simulink model "quadcopter_final"  (R2017a)
settings: Solver=VariableStepAuto  StartTime=0.0  StopTime=100  RelTol=1e-3
model workspace (MAT data in the model file):
  Izz = 0.019
values from neighbouring files (symbols this model uses):
  Ax = 0.1    [quadcopter_final.mat]
  Ay = 0.1    [quadcopter_final.mat]
  Az = 0    [quadcopter_final.mat]
  b = 3.59e-05    [quadcopter_final.mat]
  d = 2.081e-06    [quadcopter_final.mat]
  g = 9.8    [quadcopter_final.mat]
  Ixx = 0.00963    [quadcopter_final.mat]
  Iyy = 0.0096    [quadcopter_final.mat]
  Jr = 0.04439    [quadcopter_final.mat]
  l = 0.24    [quadcopter_final.mat]
  m = 0.9928    [quadcopter_final.mat]
libraries: simulink x5
settings Model: Creator=Sarthak  LastModifiedBy=Sarthak

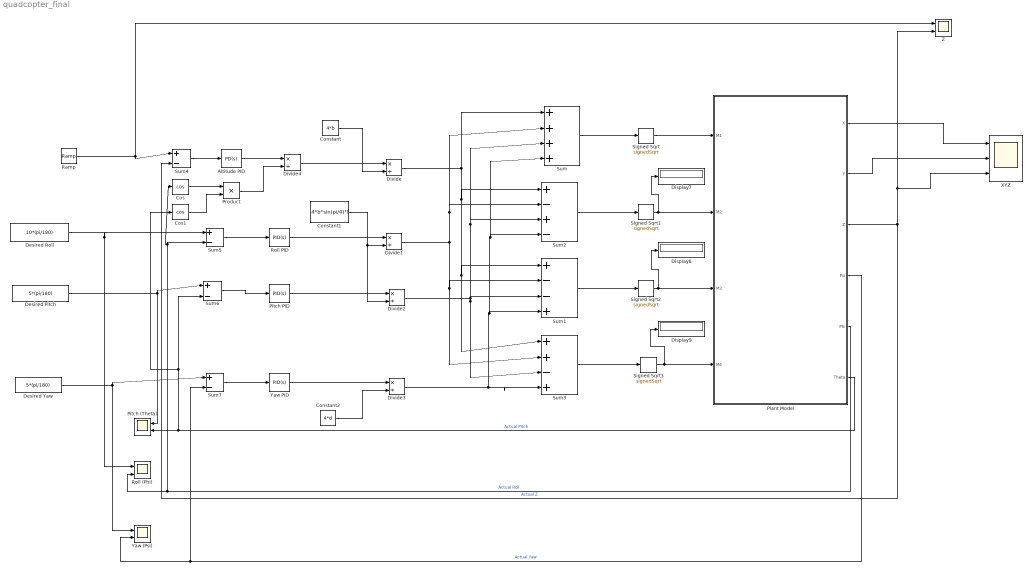
== system quadcopter_final ==
  Altitude PID : simulink/Continuous/PID Controller  Controller=PD  TimeDomain=Continuous-time  SampleTime=-1  IntegratorMethod=Forward Euler  FilterMethod=Forward Euler  Form=Parallel  UseFilter=on  ControllerParametersSource=internal  P=4  I=0.1  D=2  N=1  InitialConditionSource=internal  InitialConditionForIntegrator=0  InitialConditionForFilter=0  ExternalReset=none  LimitOutput=off  UpperSaturationLimit=inf  LowerSaturationLimit=-inf  LinearizeAsGain=on  AntiWindupMode=none  Kb=1  TrackingMode=off  Kt=1  PParamMin=[]  PParamMax=[]  IParamMin=[]  IParamMax=[]  DParamMin=[]  DParamMax=[]  NParamMin=[]  NParamMax=[]  KbParamMin=[]  KbParamMax=[]  KtParamMin=[]  KtParamMax=[]  POutMin=[]  POutMax=[]  IOutMin=[]  IOutMax=[]  DOutMin=[]  DOutMax=[]  NOutMin=[]  NOutMax=[]  KbOutMin=[]  KbOutMax=[]  KtOutMin=[]  KtOutMax=[]  IntegratorOutMin=[]  IntegratorOutMax=[]  FilterOutMin=[]  FilterOutMax=[]  SumOutMin=[]  SumOutMax=[]  SumI1OutMin=[]  SumI1OutMax=[]  SumI2OutMin=[]  SumI2OutMax=[]  SumI3OutMin=[]  SumI3OutMax=[]  SumDOutMin=[]  SumDOutMax=[]  SaturationOutMin=[]  SaturationOutMax=[]  IntegratorContinuousStateAttributes=''  IntegratorStateMustResolveToSignalObject=off  IntegratorRTWStateStorageClass=Auto  FilterContinuousStateAttributes=''  FilterStateMustResolveToSignalObject=off  FilterRTWStateStorageClass=Auto  DifferentiatorICPrevScaledInput=0  DifferentiatorOutMin=[]  DifferentiatorOutMax=[]  InitialConditionSetting=State (most efficient)
  Constant : Constant  Value=4*b
  Constant1 : Constant  Value=4*b*sin(pi/4)*l
  Constant2 : Constant  Value=4*d
  Cos : Trigonometry  Operator=cos
  Cos1 : Trigonometry  Operator=cos
  Desired Pitch : Constant  Value=5*(pi/180)
  Desired Roll : Constant  Value=10*(pi/180)
  Desired Yaw : Constant  Value=5*(pi/180)
  Display7 : Display
  Display8 : Display
  Display9 : Display
  Divide{,1..4} (5 alike) : Product  Inputs=*/
  Pitch (Theta) : Scope  NumInputPorts=2
  Pitch PID : simulink/Continuous/PID Controller  Controller=PID  TimeDomain=Continuous-time  SampleTime=-1  IntegratorMethod=Forward Euler  FilterMethod=Forward Euler  Form=Parallel  UseFilter=on  ControllerParametersSource=internal  P=1e-3  I=1e-5  D=1e-2  N=1  InitialConditionSource=internal  InitialConditionForIntegrator=0  InitialConditionForFilter=0  ExternalReset=none  LimitOutput=off  UpperSaturationLimit=inf  LowerSaturationLimit=-inf  LinearizeAsGain=on  AntiWindupMode=none  Kb=1  TrackingMode=off  Kt=1  PParamMin=[]  PParamMax=[]  IParamMin=[]  IParamMax=[]  DParamMin=[]  DParamMax=[]  NParamMin=[]  NParamMax=[]  KbParamMin=[]  KbParamMax=[]  KtParamMin=[]  KtParamMax=[]  POutMin=[]  POutMax=[]  IOutMin=[]  IOutMax=[]  DOutMin=[]  DOutMax=[]  NOutMin=[]  NOutMax=[]  KbOutMin=[]  KbOutMax=[]  KtOutMin=[]  KtOutMax=[]  IntegratorOutMin=[]  IntegratorOutMax=[]  FilterOutMin=[]  FilterOutMax=[]  SumOutMin=[]  SumOutMax=[]  SumI1OutMin=[]  SumI1OutMax=[]  SumI2OutMin=[]  SumI2OutMax=[]  SumI3OutMin=[]  SumI3OutMax=[]  SumDOutMin=[]  SumDOutMax=[]  SaturationOutMin=[]  SaturationOutMax=[]  IntegratorContinuousStateAttributes=''  IntegratorStateMustResolveToSignalObject=off  IntegratorRTWStateStorageClass=Auto  FilterContinuousStateAttributes=''  FilterStateMustResolveToSignalObject=off  FilterRTWStateStorageClass=Auto  DifferentiatorICPrevScaledInput=0  DifferentiatorOutMin=[]  DifferentiatorOutMax=[]  InitialConditionSetting=State (most efficient)
  Plant Model : Subsystem
  Product : Product
  Ramp : simulink/Sources/Ramp  slope=1  start=0  X0=0
  Roll (Phi) : Scope  NumInputPorts=2
  Roll PID : simulink/Continuous/PID Controller  Controller=PID  TimeDomain=Continuous-time  SampleTime=-1  IntegratorMethod=Forward Euler  FilterMethod=Forward Euler  Form=Parallel  UseFilter=on  ControllerParametersSource=internal  P=1e-3  I=2.45847996540361e-05  D=1  N=100  InitialConditionSource=internal  InitialConditionForIntegrator=0  InitialConditionForFilter=0  ExternalReset=none  LimitOutput=off  UpperSaturationLimit=inf  LowerSaturationLimit=-inf  LinearizeAsGain=on  AntiWindupMode=none  Kb=1  TrackingMode=off  Kt=1  PParamMin=[]  PParamMax=[]  IParamMin=[]  IParamMax=[]  DParamMin=[]  DParamMax=[]  NParamMin=[]  NParamMax=[]  KbParamMin=[]  KbParamMax=[]  KtParamMin=[]  KtParamMax=[]  POutMin=[]  POutMax=[]  IOutMin=[]  IOutMax=[]  DOutMin=[]  DOutMax=[]  NOutMin=[]  NOutMax=[]  KbOutMin=[]  KbOutMax=[]  KtOutMin=[]  KtOutMax=[]  IntegratorOutMin=[]  IntegratorOutMax=[]  FilterOutMin=[]  FilterOutMax=[]  SumOutMin=[]  SumOutMax=[]  SumI1OutMin=[]  SumI1OutMax=[]  SumI2OutMin=[]  SumI2OutMax=[]  SumI3OutMin=[]  SumI3OutMax=[]  SumDOutMin=[]  SumDOutMax=[]  SaturationOutMin=[]  SaturationOutMax=[]  IntegratorContinuousStateAttributes=''  IntegratorStateMustResolveToSignalObject=off  IntegratorRTWStateStorageClass=Auto  FilterContinuousStateAttributes=''  FilterStateMustResolveToSignalObject=off  FilterRTWStateStorageClass=Auto  DifferentiatorICPrevScaledInput=0  DifferentiatorOutMin=[]  DifferentiatorOutMax=[]  InitialConditionSetting=State (most efficient)
  Signed Sqrt{,1..3} (4 alike) : Sqrt  Operator=signedSqrt  SaturateOnIntegerOverflow=on
  Sum : Sum  Inputs=|++++
  Sum1 : Sum  Inputs=|+--+
  Sum2 : Sum  Inputs=|+-+-
  Sum3 : Sum  Inputs=|++-+
  Sum{4..7} (4 alike) : Sum  Inputs=|+-
  XYZ : Scope  NumInputPorts=3
  Yaw (Psi) : Scope  NumInputPorts=2
  Yaw PID : simulink/Continuous/PID Controller  Controller=PID  TimeDomain=Continuous-time  SampleTime=-1  IntegratorMethod=Forward Euler  FilterMethod=Forward Euler  Form=Parallel  UseFilter=on  ControllerParametersSource=internal  P=1e-3  I=1e-5  D=0.5e-2  N=1  InitialConditionSource=internal  InitialConditionForIntegrator=0  InitialConditionForFilter=0  ExternalReset=none  LimitOutput=off  UpperSaturationLimit=inf  LowerSaturationLimit=-inf  LinearizeAsGain=on  AntiWindupMode=none  Kb=1  TrackingMode=off  Kt=1  PParamMin=[]  PParamMax=[]  IParamMin=[]  IParamMax=[]  DParamMin=[]  DParamMax=[]  NParamMin=[]  NParamMax=[]  KbParamMin=[]  KbParamMax=[]  KtParamMin=[]  KtParamMax=[]  POutMin=[]  POutMax=[]  IOutMin=[]  IOutMax=[]  DOutMin=[]  DOutMax=[]  NOutMin=[]  NOutMax=[]  KbOutMin=[]  KbOutMax=[]  KtOutMin=[]  KtOutMax=[]  IntegratorOutMin=[]  IntegratorOutMax=[]  FilterOutMin=[]  FilterOutMax=[]  SumOutMin=[]  SumOutMax=[]  SumI1OutMin=[]  SumI1OutMax=[]  SumI2OutMin=[]  SumI2OutMax=[]  SumI3OutMin=[]  SumI3OutMax=[]  SumDOutMin=[]  SumDOutMax=[]  SaturationOutMin=[]  SaturationOutMax=[]  IntegratorContinuousStateAttributes=''  IntegratorStateMustResolveToSignalObject=off  IntegratorRTWStateStorageClass=Auto  FilterContinuousStateAttributes=''  FilterStateMustResolveToSignalObject=off  FilterRTWStateStorageClass=Auto  DifferentiatorICPrevScaledInput=0  DifferentiatorOutMin=[]  DifferentiatorOutMax=[]  InitialConditionSetting=State (most efficient)
  Z : Scope  NumInputPorts=2
  wires:
  Signed Sqrt/1 -> Plant Model/1(M1)
  Signed Sqrt1/1 -> Display7/1, Plant Model/2(M2)
  Signed Sqrt2/1 -> Display8/1, Plant Model/3(M3)
  Signed Sqrt3/1 -> Display9/1, Plant Model/4(M4)
  Sum/1 -> Signed Sqrt/1
  Sum2/1 -> Signed Sqrt1/1
  Sum1/1 -> Signed Sqrt2/1
  Sum3/1 -> Signed Sqrt3/1
  Divide/1 -> Sum3/1, Sum1/1, Sum2/1, Sum/1
  Divide1/1 -> Sum/2, Sum2/2, Sum3/2, Sum1/2
  Divide2/1 -> Sum3/3, Sum1/3, Sum2/3, Sum/3
  Divide3/1 -> Sum/4, Sum2/4, Sum1/4, Sum3/4
  Constant/1 -> Divide/2
  Constant1/1 -> Divide2/2, Divide1/2
  Constant2/1 -> Divide3/2
  Divide4/1 -> Divide/1
  Altitude PID/1 -> Divide4/1
  Product/1 -> Divide4/2
  Cos/1 -> Product/1
  Cos1/1 -> Product/2
  Roll PID/1 -> Divide1/1
  Pitch PID/1 -> Divide2/1
  Yaw PID/1 -> Divide3/1
  Sum4/1 -> Altitude PID/1
  Sum5/1 -> Roll PID/1
  Sum6/1 -> Pitch PID/1
  Sum7/1 -> Yaw PID/1
  Desired Roll/1 -> Roll (Phi)/1, Sum5/1
  Desired Pitch/1 -> Sum6/1, Pitch (Theta)/1
  Desired Yaw/1 -> Sum7/1, Yaw (Psi)/1
  Ramp/1 -> Sum4/1, Z/1
  Plant Model/6(Theta) -> Cos1/1, Sum6/2, Pitch (Theta)/2  "Actual Pitch"
  Plant Model/5(Phi) -> Cos/1, Sum5/2, Roll (Phi)/2  "Actual Roll"
  Plant Model/4(Psi) -> Sum7/2, Yaw (Psi)/2  "Actual Yaw"
  Plant Model/3(Z) -> Sum4/2, XYZ/3, Z/2  "Actual Z"
  Plant Model/1(X) -> XYZ/1
  Plant Model/2(Y) -> XYZ/2

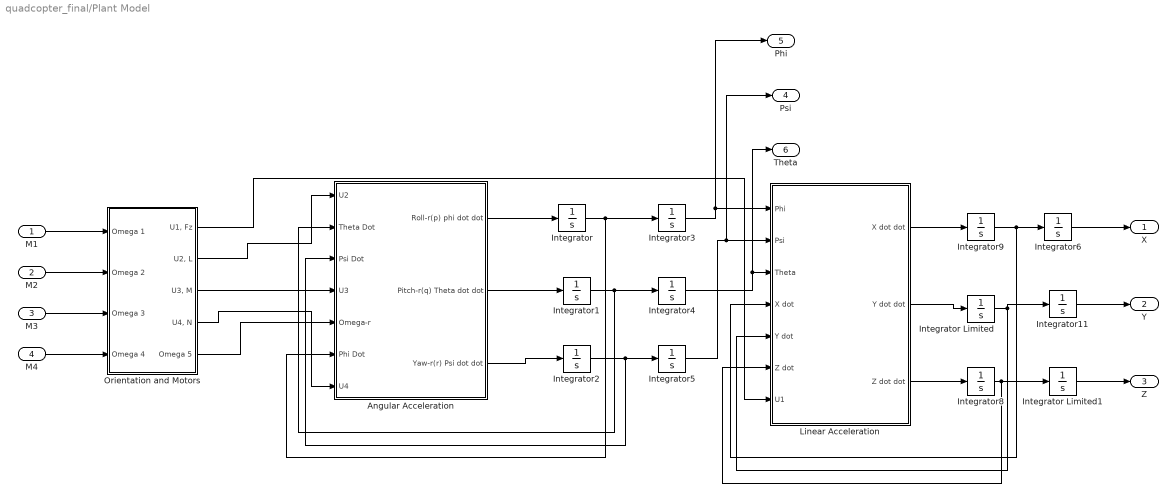
== system quadcopter_final/Plant Model ==
  M1 : Inport
  M2 : Inport  Port=2
  M3 : Inport  Port=3
  M4 : Inport  Port=4
  Angular Acceleration : Subsystem
  Integrator{,1..2,6,8..9,11} (7 alike) : Integrator
  Integrator Limited : Integrator  LimitOutput=on  LowerSaturationLimit=0
  Integrator Limited1 : Integrator  LimitOutput=on  LowerSaturationLimit=0
  Integrator3 : Integrator  WrapState=on
  Integrator4 : Integrator  WrapState=on
  Integrator5 : Integrator  WrapState=on
  Linear Acceleration : Subsystem
  Orientation and Motors : Subsystem
  X : Outport
  Y : Outport  Port=2
  Z : Outport  Port=3
  Psi : Outport  Port=4
  Phi : Outport  Port=5
  Theta : Outport  Port=6
  wires:
  M1/1 -> Orientation and Motors/1(Omega 1)
  M2/1 -> Orientation and Motors/2(Omega 2)
  M3/1 -> Orientation and Motors/3(Omega 3)
  M4/1 -> Orientation and Motors/4(Omega 4)
  Orientation and Motors/2("U2, L") -> Angular Acceleration/1(U2)
  Orientation and Motors/3("U3, M") -> Angular Acceleration/4(U3)
  Orientation and Motors/4("U4, N") -> Angular Acceleration/7(U4)
  Orientation and Motors/5(Omega 5) -> Angular Acceleration/5(Omega-r)
  Angular Acceleration/1(Roll-r(p) phi dot dot) -> Integrator/1
  Angular Acceleration/2(Pitch-r(q) Theta dot dot) -> Integrator1/1
  Angular Acceleration/3(Yaw-r(r) Psi dot dot) -> Integrator2/1
  Integrator/1 -> Angular Acceleration/6(Phi Dot), Integrator3/1
  Integrator2/1 -> Integrator5/1, Angular Acceleration/3(Psi Dot)
  Integrator3/1 -> Phi/1, Linear Acceleration/1(Phi)
  Integrator4/1 -> Theta/1, Linear Acceleration/3(Theta)
  Integrator5/1 -> Psi/1, Linear Acceleration/2(Psi)
  Integrator1/1 -> Integrator4/1, Angular Acceleration/2(Theta Dot)
  Orientation and Motors/1("U1, Fz") -> Linear Acceleration/7(U1)
  Integrator8/1 -> Integrator Limited1/1, Linear Acceleration/6(Z dot)
  Linear Acceleration/3(Z dot dot) -> Integrator8/1
  Linear Acceleration/2(Y dot dot) -> Integrator Limited/1
  Linear Acceleration/1(X dot dot) -> Integrator9/1
  Integrator9/1 -> Linear Acceleration/4(X dot), Integrator6/1
  Integrator Limited/1 -> Integrator11/1, Linear Acceleration/5(Y dot)
  Integrator Limited1/1 -> Z/1
  Integrator11/1 -> Y/1
  Integrator6/1 -> X/1

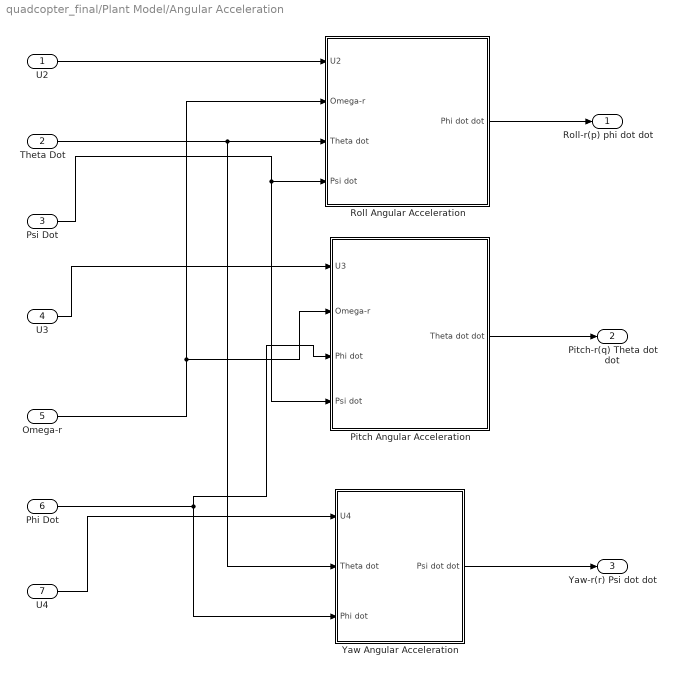
== system quadcopter_final/Plant Model/Angular Acceleration ==
  U2 : Inport
  Theta Dot : Inport  Port=2
  Psi Dot : Inport  Port=3
  U3 : Inport  Port=4
  Omega-r : Inport  Port=5
  Phi Dot : Inport  Port=6
  U4 : Inport  Port=7
  Pitch Angular Acceleration : Subsystem
  Roll Angular Acceleration : Subsystem
  Yaw Angular Acceleration : Subsystem
  Roll-r(p) phi dot dot : Outport
  Pitch-r(q) Theta dot dot : Outport  Port=2
  Yaw-r(r) Psi dot dot : Outport  Port=3
  wires:
  U2/1 -> Roll Angular Acceleration/1(U2)
  Omega-r/1 -> Pitch Angular Acceleration/2(Omega-r), Roll Angular Acceleration/2(Omega-r)
  Theta Dot/1 -> Yaw Angular Acceleration/2(Theta dot), Roll Angular Acceleration/3(Theta dot)
  Psi Dot/1 -> Pitch Angular Acceleration/4(Psi dot), Roll Angular Acceleration/4(Psi dot)
  U3/1 -> Pitch Angular Acceleration/1(U3)
  Phi Dot/1 -> Pitch Angular Acceleration/3(Phi dot), Yaw Angular Acceleration/3(Phi dot)
  U4/1 -> Yaw Angular Acceleration/1(U4)
  Roll Angular Acceleration/1(Phi dot dot) -> Roll-r(p) phi dot dot/1
  Pitch Angular Acceleration/1(Theta dot dot) -> Pitch-r(q) Theta dot dot/1
  Yaw Angular Acceleration/1(Psi dot dot) -> Yaw-r(r) Psi dot dot/1

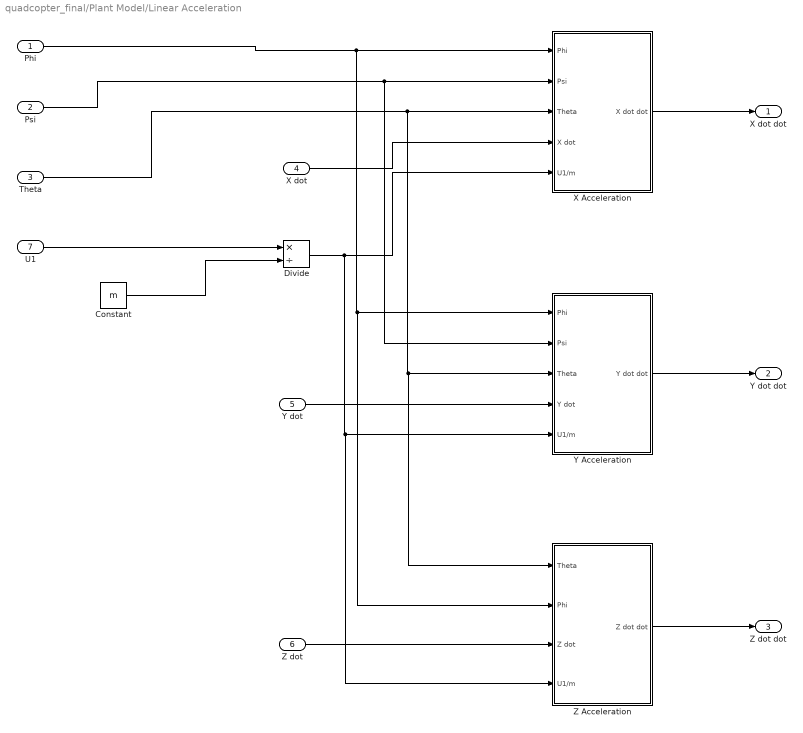
== system quadcopter_final/Plant Model/Linear Acceleration ==
  Phi : Inport
  Psi : Inport  Port=2
  Theta : Inport  Port=3
  X dot : Inport  Port=4
  Y dot : Inport  Port=5
  Z dot : Inport  Port=6
  U1 : Inport  Port=7
  Constant : Constant  Value=m
  Divide : Product  Inputs=*/
  X Acceleration : Subsystem
  Y Acceleration : Subsystem
  Z Acceleration : Subsystem
  X dot dot : Outport
  Y dot dot : Outport  Port=2
  Z dot dot : Outport  Port=3
  wires:
  Phi/1 -> Z Acceleration/2(Phi), Y Acceleration/1(Phi), X Acceleration/1(Phi)
  Psi/1 -> Y Acceleration/2(Psi), X Acceleration/2(Psi)
  Theta/1 -> Z Acceleration/1(Theta), Y Acceleration/3(Theta), X Acceleration/3(Theta)
  X dot/1 -> X Acceleration/4(X dot)
  Divide/1 -> Z Acceleration/4(U1/m), Y Acceleration/5(U1/m), X Acceleration/5(U1/m)
  U1/1 -> Divide/1
  Constant/1 -> Divide/2
  X Acceleration/1(X dot dot) -> X dot dot/1
  Y dot/1 -> Y Acceleration/4(Y dot)
  Y Acceleration/1(Y dot dot) -> Y dot dot/1
  Z dot/1 -> Z Acceleration/3(Z dot)
  Z Acceleration/1(Z dot dot) -> Z dot dot/1

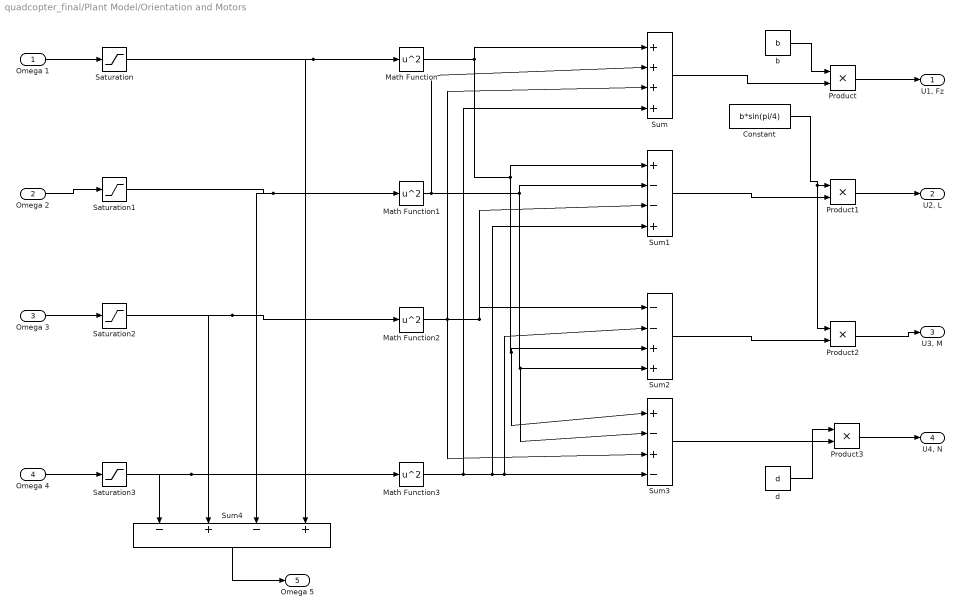
== system quadcopter_final/Plant Model/Orientation and Motors ==
  Omega 1 : Inport
  Omega 2 : Inport  Port=2
  Omega 3 : Inport  Port=3
  Omega 4 : Inport  Port=4
  Constant : Constant  Value=b*sin(pi/4)
  Math Function{,1..3} (4 alike) : Math  Operator=square  SaturateOnIntegerOverflow=on
  Product{,1..3} (4 alike) : Product
  Saturation{,1..3} (4 alike) : Saturate  UpperLimit=inf  LowerLimit=0
  Sum : Sum  Inputs=|++++
  Sum1 : Sum  Inputs=|+--+
  Sum2 : Sum  Inputs=|--++
  Sum3 : Sum  Inputs=|+-+-
  Sum4 : Sum  Inputs=|-+-+
  "b " : Constant  Value=b
  d : Constant  Value=d
  "U1, Fz" : Outport
  "U2, L" : Outport  Port=2
  "U3, M" : Outport  Port=3
  "U4, N" : Outport  Port=4
  Omega 5 : Outport  Port=5
  wires:
  Product/1 -> "U1, Fz"/1
  Product1/1 -> "U2, L"/1
  Product2/1 -> "U3, M"/1
  Product3/1 -> "U4, N"/1
  Sum/1 -> Product/2
  Sum1/1 -> Product1/2
  Sum2/1 -> Product2/2
  Sum3/1 -> Product3/2
  "b "/1 -> Product/1
  d/1 -> Product3/1
  Constant/1 -> Product1/1, Product2/1
  Math Function/1 -> Sum3/1, Sum2/3, Sum1/1, Sum/1
  Math Function1/1 -> Sum/2, Sum3/2, Sum2/4, Sum1/2
  Math Function2/1 -> Sum3/3, Sum/3, Sum1/3, Sum2/1
  Math Function3/1 -> Sum/4, Sum1/4, Sum2/2, Sum3/4
  Omega 1/1 -> Saturation/1
  Saturation/1 -> Sum4/4, Math Function/1
  Saturation1/1 -> Sum4/3, Math Function1/1
  Saturation2/1 -> Sum4/2, Math Function2/1
  Saturation3/1 -> Sum4/1, Math Function3/1
  Omega 4/1 -> Saturation3/1
  Omega 3/1 -> Saturation2/1
  Omega 2/1 -> Saturation1/1
  Sum4/1 -> Omega 5/1

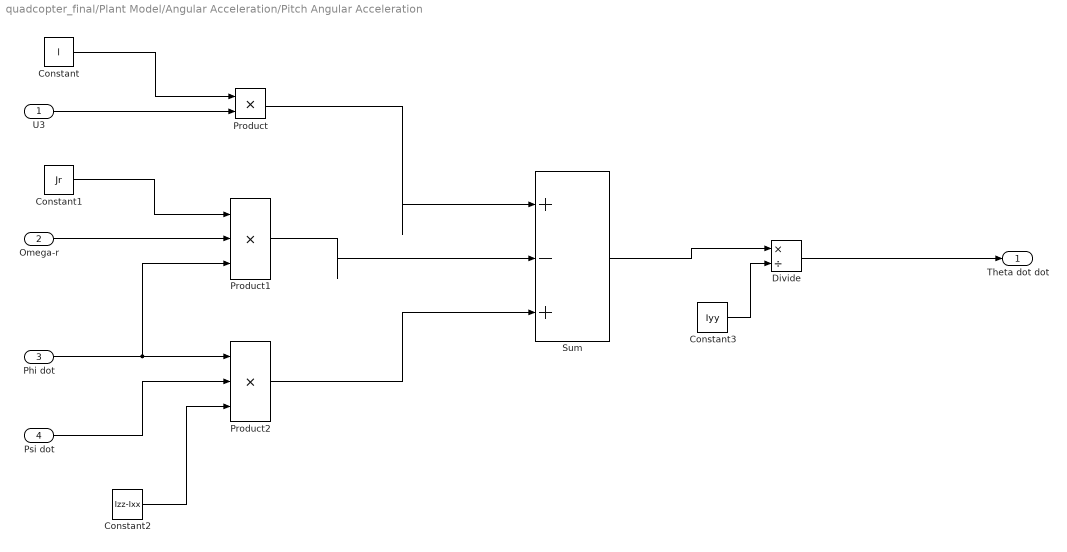
== system quadcopter_final/Plant Model/Angular Acceleration/Pitch Angular Acceleration ==
  U3 : Inport
  Omega-r : Inport  Port=2
  Phi dot : Inport  Port=3
  Psi dot : Inport  Port=4
  Constant : Constant  Value=l
  Constant1 : Constant  Value=Jr
  Constant2 : Constant  Value=Izz-Ixx
  Constant3 : Constant  Value=Iyy
  Divide : Product  Inputs=*/
  Product : Product
  Product1 : Product  Inputs=3
  Product2 : Product  Inputs=3
  Sum : Sum  Inputs=|+-+
  Theta dot dot : Outport
  wires:
  U3/1 -> Product/2
  Constant/1 -> Product/1
  Omega-r/1 -> Product1/2
  Constant1/1 -> Product1/1
  Phi dot/1 -> Product2/1, Product1/3
  Psi dot/1 -> Product2/2
  Constant2/1 -> Product2/3
  Product/1 -> Sum/1
  Product1/1 -> Sum/2
  Product2/1 -> Sum/3
  Sum/1 -> Divide/1
  Constant3/1 -> Divide/2
  Divide/1 -> Theta dot dot/1

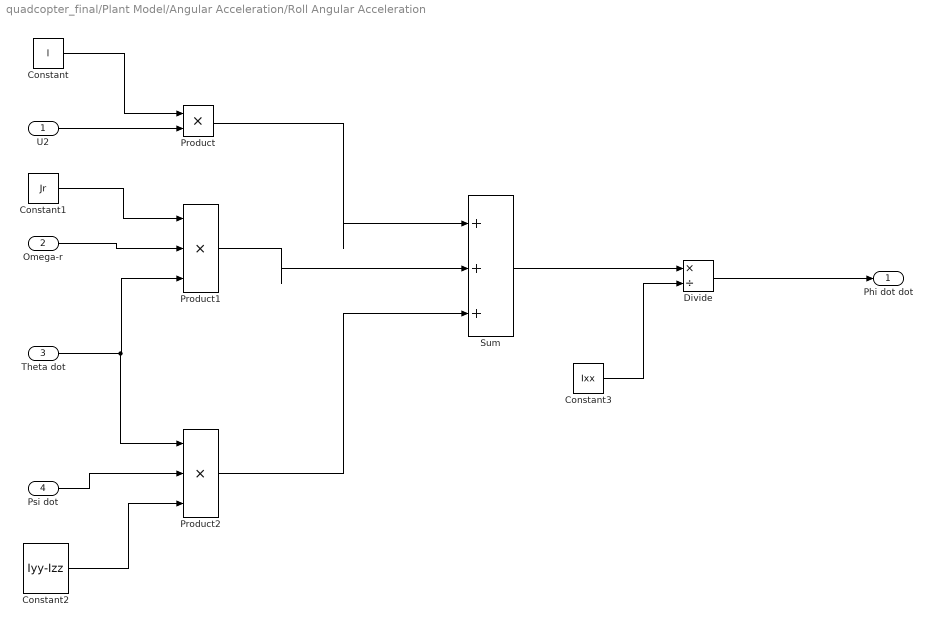
== system quadcopter_final/Plant Model/Angular Acceleration/Roll Angular Acceleration ==
  U2 : Inport
  Omega-r : Inport  Port=2
  Theta dot : Inport  Port=3
  Psi dot : Inport  Port=4
  Constant : Constant  Value=l
  Constant1 : Constant  Value=Jr
  Constant2 : Constant  Value=Iyy-Izz
  Constant3 : Constant  Value=Ixx
  Divide : Product  Inputs=*/
  Product : Product
  Product1 : Product  Inputs=3
  Product2 : Product  Inputs=3
  Sum : Sum  Inputs=|+++
  Phi dot dot : Outport
  wires:
  Constant/1 -> Product/1
  U2/1 -> Product/2
  Constant1/1 -> Product1/1
  Omega-r/1 -> Product1/2
  Theta dot/1 -> Product2/1, Product1/3
  Psi dot/1 -> Product2/2
  Constant2/1 -> Product2/3
  Product/1 -> Sum/1
  Product1/1 -> Sum/2
  Product2/1 -> Sum/3
  Sum/1 -> Divide/1
  Constant3/1 -> Divide/2
  Divide/1 -> Phi dot dot/1

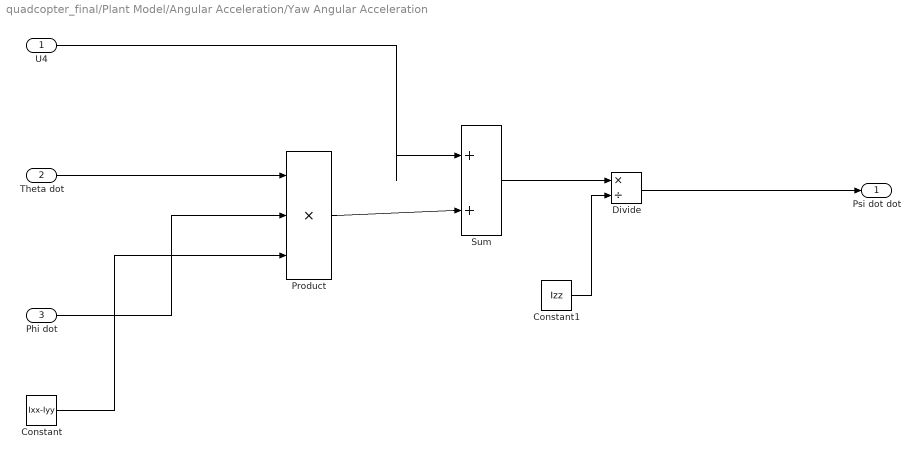
== system quadcopter_final/Plant Model/Angular Acceleration/Yaw Angular Acceleration ==
  U4 : Inport
  Theta dot : Inport  Port=2
  Phi dot : Inport  Port=3
  Constant : Constant  Value=Ixx-Iyy
  Constant1 : Constant  Value=Izz
  Divide : Product  Inputs=*/
  Product : Product  Inputs=3
  Sum : Sum  Inputs=|++
  Psi dot dot : Outport
  wires:
  Theta dot/1 -> Product/1
  Phi dot/1 -> Product/2
  Constant/1 -> Product/3
  Product/1 -> Sum/2
  U4/1 -> Sum/1
  Sum/1 -> Divide/1
  Constant1/1 -> Divide/2
  Divide/1 -> Psi dot dot/1

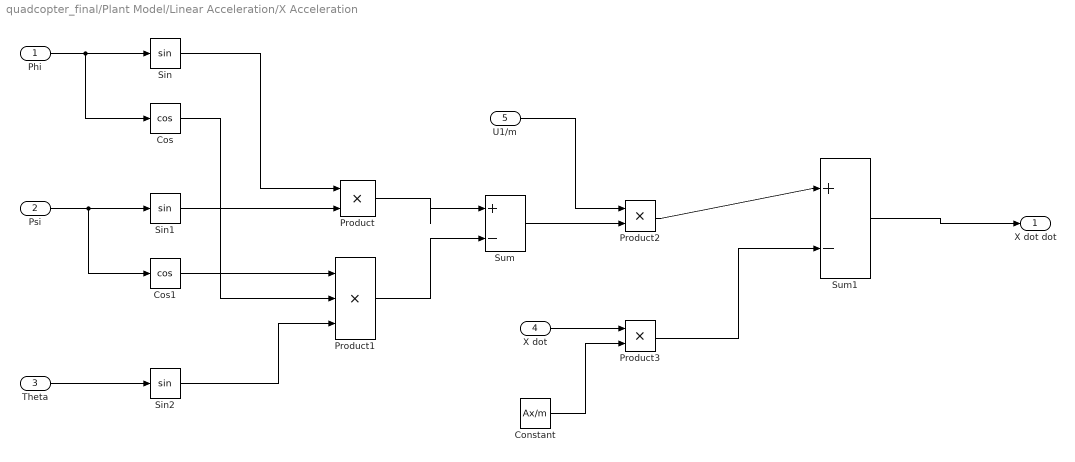
== system quadcopter_final/Plant Model/Linear Acceleration/X Acceleration ==
  Phi : Inport
  Psi : Inport  Port=2
  Theta : Inport  Port=3
  X dot : Inport  Port=4
  U1/m : Inport  Port=5
  Constant : Constant  Value=Ax/m
  Cos : Trigonometry  Operator=cos
  Cos1 : Trigonometry  Operator=cos
  Product : Product
  Product1 : Product  Inputs=3
  Product2 : Product
  Product3 : Product
  Sin : Trigonometry
  Sin1 : Trigonometry
  Sin2 : Trigonometry
  Sum : Sum  Inputs=|+-
  Sum1 : Sum  Inputs=|+-
  X dot dot : Outport
  wires:
  Phi/1 -> Cos/1, Sin/1
  Psi/1 -> Cos1/1, Sin1/1
  Theta/1 -> Sin2/1
  Sin1/1 -> Product/2
  Sin/1 -> Product/1
  Cos1/1 -> Product1/1
  Cos/1 -> Product1/2
  Sin2/1 -> Product1/3
  Product/1 -> Sum/1
  Product1/1 -> Sum/2
  Sum/1 -> Product2/2
  U1/m/1 -> Product2/1
  X dot/1 -> Product3/1
  Constant/1 -> Product3/2
  Product2/1 -> Sum1/1
  Product3/1 -> Sum1/2
  Sum1/1 -> X dot dot/1

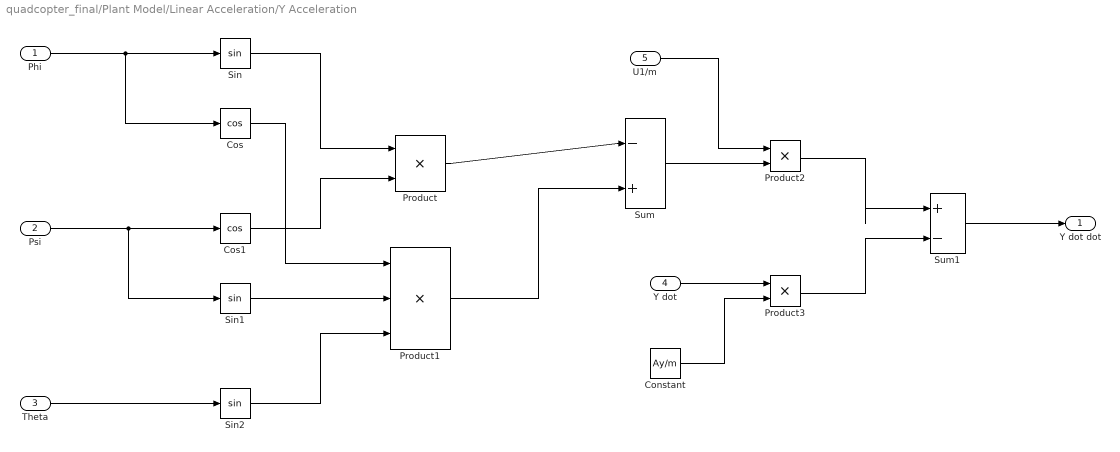
== system quadcopter_final/Plant Model/Linear Acceleration/Y Acceleration ==
  Phi : Inport
  Psi : Inport  Port=2
  Theta : Inport  Port=3
  Y dot : Inport  Port=4
  U1/m : Inport  Port=5
  Constant : Constant  Value=Ay/m
  Cos : Trigonometry  Operator=cos
  Cos1 : Trigonometry  Operator=cos
  Product : Product
  Product1 : Product  Inputs=3
  Product2 : Product
  Product3 : Product
  Sin : Trigonometry
  Sin1 : Trigonometry
  Sin2 : Trigonometry
  Sum : Sum  Inputs=|-+
  Sum1 : Sum  Inputs=|+-
  Y dot dot : Outport
  wires:
  Phi/1 -> Cos/1, Sin/1
  Psi/1 -> Sin1/1, Cos1/1
  Theta/1 -> Sin2/1
  Sin/1 -> Product/1
  Cos1/1 -> Product/2
  Cos/1 -> Product1/1
  Sin1/1 -> Product1/2
  Sin2/1 -> Product1/3
  Product/1 -> Sum/1
  Product1/1 -> Sum/2
  Sum/1 -> Product2/2
  U1/m/1 -> Product2/1
  Y dot/1 -> Product3/1
  Constant/1 -> Product3/2
  Product2/1 -> Sum1/1
  Product3/1 -> Sum1/2
  Sum1/1 -> Y dot dot/1

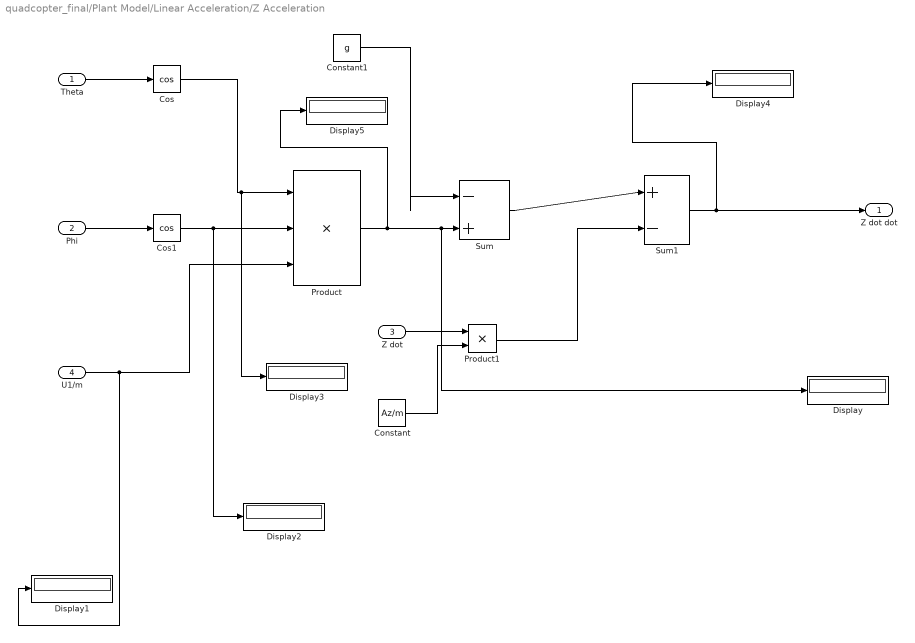
== system quadcopter_final/Plant Model/Linear Acceleration/Z Acceleration ==
  Theta : Inport
  Phi : Inport  Port=2
  Z dot : Inport  Port=3
  U1/m : Inport  Port=4
  Constant : Constant  Value=Az/m
  Constant1 : Constant  Value=g
  Cos : Trigonometry  Operator=cos
  Cos1 : Trigonometry  Operator=cos
  Display{,1..5} (6 alike) : Display
  Product : Product  Inputs=3
  Product1 : Product
  Sum : Sum  Inputs=|-+
  Sum1 : Sum  Inputs=|+-
  Z dot dot : Outport
  wires:
  Theta/1 -> Cos/1
  Phi/1 -> Cos1/1
  U1/m/1 -> Display1/1, Product/3
  Cos1/1 -> Display2/1, Product/2
  Cos/1 -> Display3/1, Product/1
  Z dot/1 -> Product1/1
  Constant/1 -> Product1/2
  Product/1 -> Display5/1, Display/1, Sum/2
  Constant1/1 -> Sum/1
  Sum/1 -> Sum1/1
  Product1/1 -> Sum1/2
  Sum1/1 -> Display4/1, Z dot dot/1
